simulink model "simulink_model_closed_loop"  (R2022a)
settings: Solver=FixedStepAuto  StartTime=0.0  StopTime=stop_time  FixedStep=T_sim  RelTol=1e-3
values from neighbouring files (symbols this model uses):
  N = 100    [nmpc_acados_setup.m]    (also in nmpc_acados_simulink_tuning.m)
  nu = 4    [nmpc_acados_setup.m]    (also in nmpc_acados_simulink_tuning.m)
  params = [params; params_i]    [nmpc_acados_setup.m]    (also in nmpc_acados_simulink_tuning.m)
  params_i = [ref; cost]    [nmpc_acados_setup.m]    (also in nmpc_acados_simulink_tuning.m)
  T_delay = 0.00    (= 0)    [nmpc_acados_simulink_test.m]    (also in nmpc_acados_simulink_tuning.m = T_delays(i))
  T_sim = 1.0/1000.0    (= 0.001)    [nmpc_acados_simulink_test.m]    (also in nmpc_acados_simulink_tuning.m)
  U_max = 1    [nmpc_acados_setup.m]    (also in nmpc_acados_simulink_tuning.m)
  x0 = [ ... (first row only)    [nmpc_acados_simulink_test.m]    (also in nmpc_acados_simulink_tuning.m)
settings Model: Creator=oj  LastModifiedBy=andreatagliabue
settings SolverCC: AlgebraicLoopSolver=TrustRegion
settings DataIOCC: SaveFormat=StructureWithTime
settings OptimizationCC: LifeSpan=inf
settings DebuggingCC: UnconnectedInputMsg=warning  UnconnectedOutputMsg=warning  UnconnectedLineMsg=warning  SFExecutionAtInitializationDiag=none  SFMachineParentedDataDiag=warning  ArithmeticOperatorsInVariantConditions=warning
settings HardwareCC: ProdBitPerSizeT=32  ProdBitPerPtrDiffT=32  ProdWordSize=32  ProdHWDeviceType=Specified
settings SFSimCC: CustomCodeUndefinedFunction=UseInterfaceOnly
settings CodeAppCC: StateflowObjectComments=on

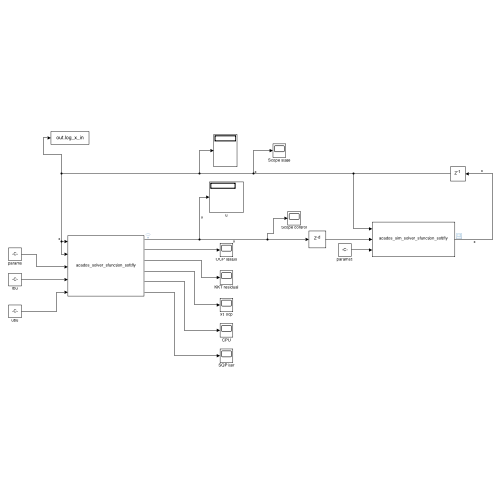
[thumbnail: Simulink's stored preview of the top-level diagram]
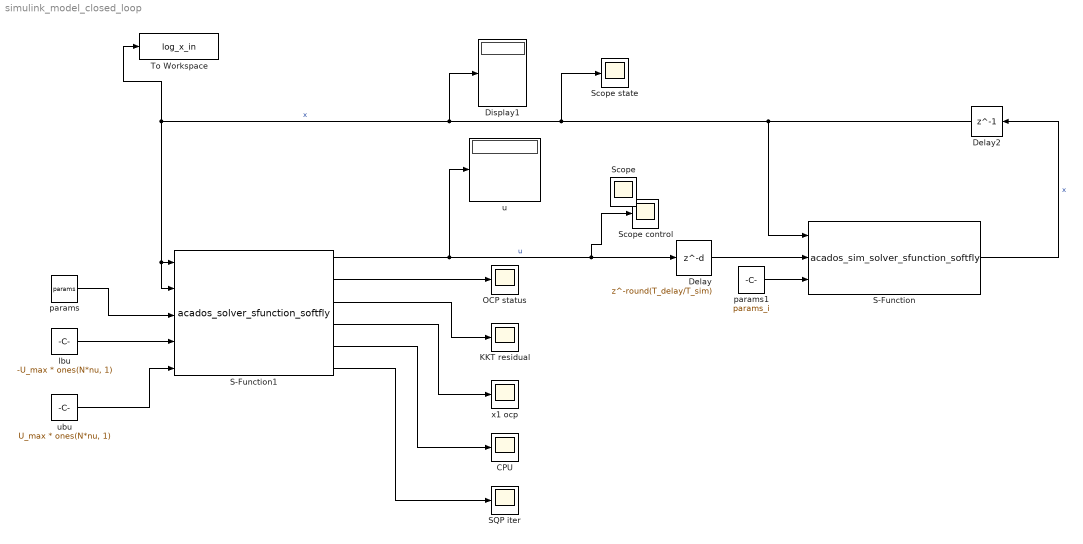
== system simulink_model_closed_loop ==
  CPU : Scope
      settings: Description=status
  Delay : Delay  DelayLength=round(T_delay/T_sim)
  Delay2 : Delay  DelayLength=1  InitialCondition=x0
  Display1 : Display
  KKT residual : Scope
      settings: Description=status
  OCP status : Scope
      settings: Description=status
  S-Function : S-Function  FunctionName=acados_sim_solver_sfunction_softfly  SFunctionDeploymentMode=off  EnableBusSupport=off
  S-Function1 : S-Function  FunctionName=acados_solver_sfunction_softfly  SFunctionDeploymentMode=off  EnableBusSupport=off
  SQP iter : Scope
      settings: Description=status
  Scope control : Scope
  Scope state : Scope
  To Workspace : ToWorkspace  VariableName=log_x_in  SaveFormat=Timeseries  SampleTime=-1
  lbu : Constant  Value=-U_max * ones(N*nu, 1)
  params : Constant  Value=params
  params1 : Constant  Value=params_i
  u : Display
  ubu : Constant  Value=U_max * ones(N*nu, 1)
  x1 ocp : Scope
      settings: Description=status
  Scope : Scope
  wires:
  S-Function/1 -> Delay2/1  "x"
  S-Function1/2 -> OCP status/1
  S-Function1/3 -> KKT residual/1
  S-Function1/4 -> x1 ocp/1
  S-Function1/5 -> CPU/1
  S-Function1/1 -> u/1, Scope control/1, Delay/1  "u"
  S-Function1/6 -> SQP iter/1
  lbu/1 -> S-Function1/4
  ubu/1 -> S-Function1/5
  params/1 -> S-Function1/3
  params1/1 -> S-Function/3
  Delay/1 -> S-Function/2
  Delay2/1 -> S-Function/1, S-Function1/2, S-Function1/1, To Workspace/1, Display1/1, Scope state/1  "x"
